simulink model "hvac_maborrelli_singapur_nzones_TCH"  (R2021a)
settings: Solver=ode45  StartTime=0.0  StopTime=Inf  FixedStep=2  RelTol=1e-3  EnableMultiTasking=on
values from neighbouring files (symbols this model uses):
  beta = 0.15    [main_td3_nzones.m]
  ci = ci'    [localResetFcn.m]    (also in localResetFcnT.m)
  CO2_max = 1200*1e-6    (= 0.0012)    [main_td3_nzones.m]
  high = 25    [main_td3_nzones.m]    (also in reward.m)
  low = -10    [isDone.m]    (also in main_td3_nzones.m = 22; reward.m = 22)
  params = params1    [main_td3_nzones.m]
  paramsnz =     [values4z_tch.mat]
  Ts = delta*Tr+(1-delta)*Toa + DT + DTH    [dynamics_hvac_maborrelli_singapur_1zone_tch.m]    (also in main_td3_nzones.m = 60)
  Ts2 = 900    [main.m]    (also in main_td3_nzones.m = 600)
undefined symbols (not defined in the file or in its folder): id, rl
libraries: simulink x15, dspmathops x5, rllib x1
settings Model: Creator=User  LastModifiedBy=Richi
settings SolverCC: AlgebraicLoopSolver=TrustRegion
settings DataIOCC: LimitDataPoints=on  SaveFormat=Array  SignalLoggingSaveFormat=ModelDataLogs
settings OptimizationCC: LifeSpan=inf
settings DebuggingCC: SolverPrmCheckMsg=warning  MultiTaskDSMMsg=warning  MultiTaskCondExecSysMsg=none  MultiTaskRateTransMsg=warning  StrictBusMsg=ErrorOnBusTreatedAsVector  SFUnexpectedBacktrackingDiag=warning  SFNoUnconditionalDefaultTransitionDiag=warning  SFExecutionAtInitializationDiag=none  SFMachineParentedDataDiag=warning  ArithmeticOperatorsInVariantConditions=warning
settings HardwareCC: ProdBitPerPointer=32  ProdBitPerSizeT=32  ProdBitPerPtrDiffT=32  ProdLargestAtomicFloat=None  ProdIntDivRoundTo=Undefined  ProdEndianess=Unspecified  ProdWordSize=32  ProdHWDeviceType=32-bit Generic
settings ModelReferenceCC: PropagateSignalLabelsOutOfModel=off
settings SFSimCC: SimUseLocalCustomCode=off  CustomCodeUndefinedFunction=UseInterfaceOnly
settings RTWCC: RTWUseLocalCustomCode=off
settings CodeAppCC: StateflowObjectComments=on
settings GRTTargetCC: TargetLangStandard=C89/C90 (ANSI)
settings ConfigComp: CovMetricSettings=dw  CovSaveCumulativeToWorkspaceVar=on  CovSaveSingleToWorkspaceVar=on  CovExternalEMLEnable=off

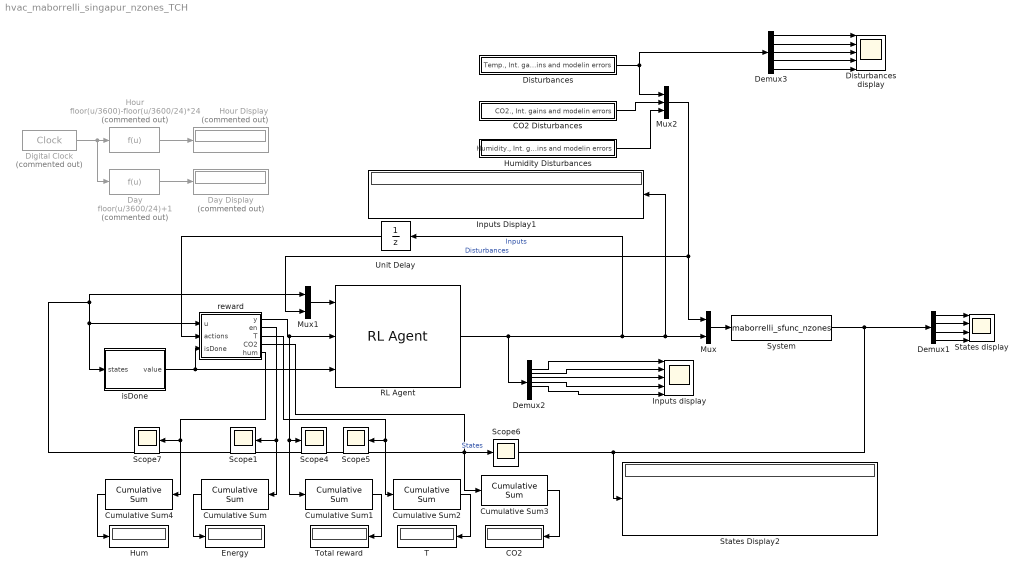
== system hvac_maborrelli_singapur_nzones_TCH ==
  CO2 : Display
  CO2 Disturbances : Subsystem  TreatAsAtomicUnit=on
  Cumulative Sum{,1..4} (5 alike) : dspmathops/Cumulative Sum  dim=Channels (running sum)  InputProcessing=Columns as channels (frame based)  reset_popup=None  roundingMode=Floor  overflowMode=off  outputDataTypeStr=Inherit: Same as accumulator  outputMin=[]  outputMax=[]  outputLastDataTypeStr=Inherit: Same as accumulator
  Day : Fcn  Commented=on  Expr=floor(u/3600/24)+1  SampleTime=1800
  Day Display : Display  Commented=on
  Demux1 : Demux
  Demux2 : Demux  Outputs=6
  Demux3 : Demux  Outputs=5
  Digital Clock : DigitalClock  Commented=on  SampleTime=60
  Disturbances : Subsystem  TreatAsAtomicUnit=on
  Disturbances display : Scope  NumInputPorts=5
  Energy : Display
  Hour : Fcn  Commented=on  Expr=floor(u/3600)-floor(u/3600/24)*24  SampleTime=1800
  Hour Display : Display  Commented=on
  Hum : Display
  Humidity Disturbances : Subsystem  TreatAsAtomicUnit=on
  Inputs Display1 : Display
  Inputs display : Scope  NumInputPorts=5
  Mux : Mux  Inputs=2
  Mux1 : Mux  Inputs=2
  Mux2 : Mux  Inputs=3
  RL Agent : rllib/RL Agent  Agent=rl.util.PolicyInstance.get('hvac_maborrelli_singapur_nzones_with_MPC_v3_manualdist_3/RL Agent')  ExternalActionAsInput=off  ProvideCumRwd=off  TreatAsDirectFeedthrough=on
  Scope{1,4..7} (5 alike) : Scope
  States Display2 : Display
  States display : Scope  NumInputPorts=4
  System : S-Function  FunctionName=maborrelli_sfunc_nzones  Parameters=ci,paramsnz,Ts  SFunctionDeploymentMode=off  EnableBusSupport=off
  T : Display
  Total reward : Display
  Unit Delay : UnitDelay  SampleTime=Ts2  HasFrameUpgradeWarning=on
  isDone : MATLAB Function  TreatAsAtomicUnit=on
  reward : MATLAB Function  TreatAsAtomicUnit=on
  wires:
  Mux/1 -> System/1
  System/1 -> Demux1/1, States Display2/1, Mux1/1, isDone/1(states), reward/1(u)  "States"
  RL Agent/1 -> Unit Delay/1, Mux/2, Inputs Display1/1, Demux2/1  "Inputs"
  Hour/1 -> Hour Display/1
  Digital Clock/1 -> Day/1, Hour/1
  Day/1 -> Day Display/1
  Demux1/1 -> States display/1
  Demux1/2 -> States display/2
  Demux1/3 -> States display/3
  Demux1/4 -> States display/4
  Demux2/1 -> Inputs display/1
  Demux2/2 -> Inputs display/2
  Demux2/3 -> Inputs display/3
  Demux2/4 -> Inputs display/4
  Demux2/5 -> Inputs display/5
  isDone/1(value) -> reward/3(isDone), RL Agent/3
  Mux1/1 -> RL Agent/1
  Unit Delay/1 -> reward/2(actions)
  Disturbances/1("Temp., Int. gains and modelin errors") -> Mux2/1, Demux3/1
  CO2 Disturbances/1("CO2., Int. gains and modelin errors") -> Mux2/2
  Humidity Disturbances/1("Humidity., Int. gains and modelin errors") -> Mux2/3
  Mux2/1 -> Mux1/2, Mux/1  "Disturbances"
  Demux3/1 -> Disturbances display/1
  Cumulative Sum4/1 -> Hum/1
  reward/4(CO2) -> Cumulative Sum3/1, Scope6/1
  Cumulative Sum/1 -> Energy/1
  Cumulative Sum2/1 -> T/1
  reward/5(hum) -> Cumulative Sum4/1, Scope7/1
  Cumulative Sum3/1 -> CO2/1
  reward/1(y) -> Cumulative Sum1/1, Scope4/1, RL Agent/2
  reward/3(T) -> Cumulative Sum2/1, Scope5/1
  Cumulative Sum1/1 -> Total reward/1
  reward/2(en) -> Cumulative Sum/1, Scope1/1
  Demux3/2 -> Disturbances display/2
  Demux3/3 -> Disturbances display/3
  Demux3/4 -> Disturbances display/4
  Demux3/5 -> Disturbances display/5

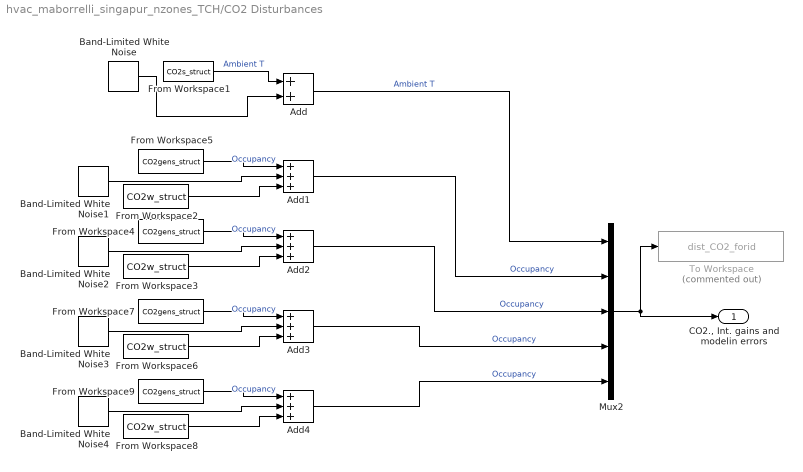
== system hvac_maborrelli_singapur_nzones_TCH/CO2 Disturbances ==
  Add : Sum
  Add{1..4} (4 alike) : Sum  Inputs=+++
  Band-Limited White Noise{,1..4} (5 alike) : simulink/Sources/Band-Limited White Noise  Cov=0  Ts=Ts  seed=[23341]
  From Workspace1 : FromWorkspace  VariableName=CO2s_struct  OutDataTypeStr=double  SampleTime=Ts  ZeroCross=off
  From Workspace{2..3,6,8} (4 alike) : FromWorkspace  VariableName=CO2w_struct  OutDataTypeStr=double  SampleTime=Ts  ZeroCross=off
  From Workspace{4..5,7,9} (4 alike) : FromWorkspace  VariableName=CO2gens_struct  OutDataTypeStr=double  SampleTime=Ts  ZeroCross=off
  Mux2 : Mux  Inputs=5
  To Workspace : ToWorkspace  Commented=on  VariableName=dist_CO2_forid  SaveFormat=Timeseries  SampleTime=id.Delta
  "CO2., Int. gains and modelin errors" : Outport
  wires:
  From Workspace1/1 -> Add/1  "Ambient T"
  Band-Limited White Noise/1 -> Add/2
  Add/1 -> Mux2/1  "Ambient T"
  From Workspace5/1 -> Add1/1  "Occupancy"
  Band-Limited White Noise1/1 -> Add1/2
  From Workspace2/1 -> Add1/3
  Mux2/1 -> "CO2., Int. gains and modelin errors"/1, To Workspace/1
  Add1/1 -> Mux2/2  "Occupancy"
  Add2/1 -> Mux2/3  "Occupancy"
  From Workspace3/1 -> Add2/3
  Band-Limited White Noise2/1 -> Add2/2
  From Workspace4/1 -> Add2/1  "Occupancy"
  Add3/1 -> Mux2/4  "Occupancy"
  From Workspace6/1 -> Add3/3
  Band-Limited White Noise3/1 -> Add3/2
  From Workspace7/1 -> Add3/1  "Occupancy"
  Add4/1 -> Mux2/5  "Occupancy"
  From Workspace8/1 -> Add4/3
  Band-Limited White Noise4/1 -> Add4/2
  From Workspace9/1 -> Add4/1  "Occupancy"

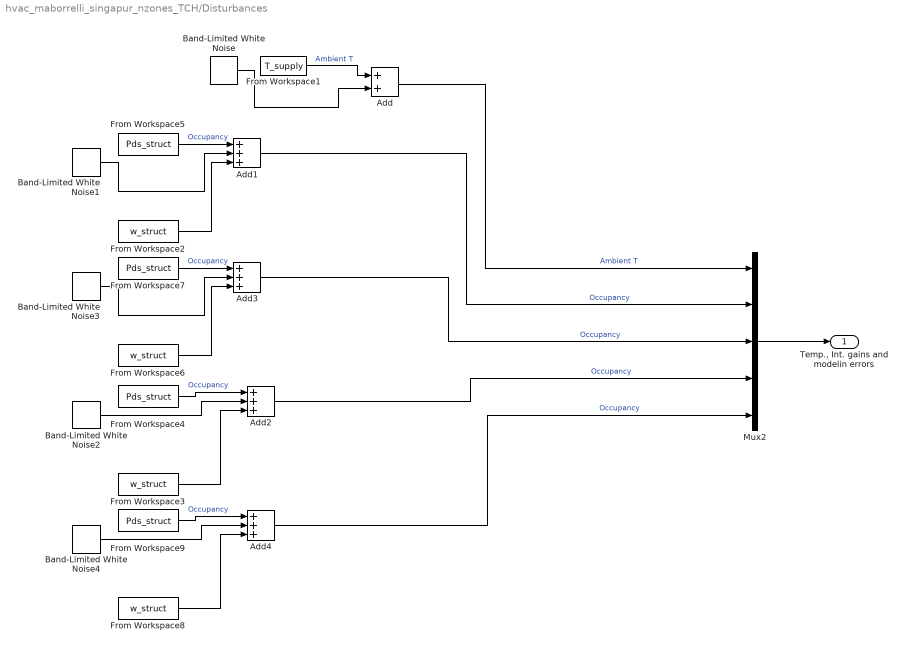
== system hvac_maborrelli_singapur_nzones_TCH/Disturbances ==
  Add : Sum
  Add{1..4} (4 alike) : Sum  Inputs=+++
  Band-Limited White Noise{,1..4} (5 alike) : simulink/Sources/Band-Limited White Noise  Cov=0  Ts=Ts2  seed=[23341]
  From Workspace1 : FromWorkspace  VariableName=T_supply  OutDataTypeStr=double  SampleTime=Ts  ZeroCross=off
  From Workspace{2..3,6,8} (4 alike) : FromWorkspace  VariableName=w_struct  OutDataTypeStr=double  SampleTime=Ts  ZeroCross=off
  From Workspace{4..5,7,9} (4 alike) : FromWorkspace  VariableName=Pds_struct  OutDataTypeStr=double  SampleTime=Ts  ZeroCross=off
  Mux2 : Mux  Inputs=5
  "Temp., Int. gains and modelin errors" : Outport
  wires:
  Add1/1 -> Mux2/2  "Occupancy"
  From Workspace1/1 -> Add/1  "Ambient T"
  Band-Limited White Noise/1 -> Add/2
  Add/1 -> Mux2/1  "Ambient T"
  From Workspace5/1 -> Add1/1  "Occupancy"
  Band-Limited White Noise1/1 -> Add1/2
  From Workspace2/1 -> Add1/3
  Mux2/1 -> "Temp., Int. gains and modelin errors"/1
  Add2/1 -> Mux2/4  "Occupancy"
  Band-Limited White Noise2/1 -> Add2/2
  From Workspace3/1 -> Add2/3
  Add3/1 -> Mux2/3  "Occupancy"
  Band-Limited White Noise3/1 -> Add3/2
  From Workspace6/1 -> Add3/3
  From Workspace7/1 -> Add3/1  "Occupancy"
  From Workspace4/1 -> Add2/1  "Occupancy"
  Add4/1 -> Mux2/5  "Occupancy"
  From Workspace8/1 -> Add4/3
  From Workspace9/1 -> Add4/1  "Occupancy"
  Band-Limited White Noise4/1 -> Add4/2

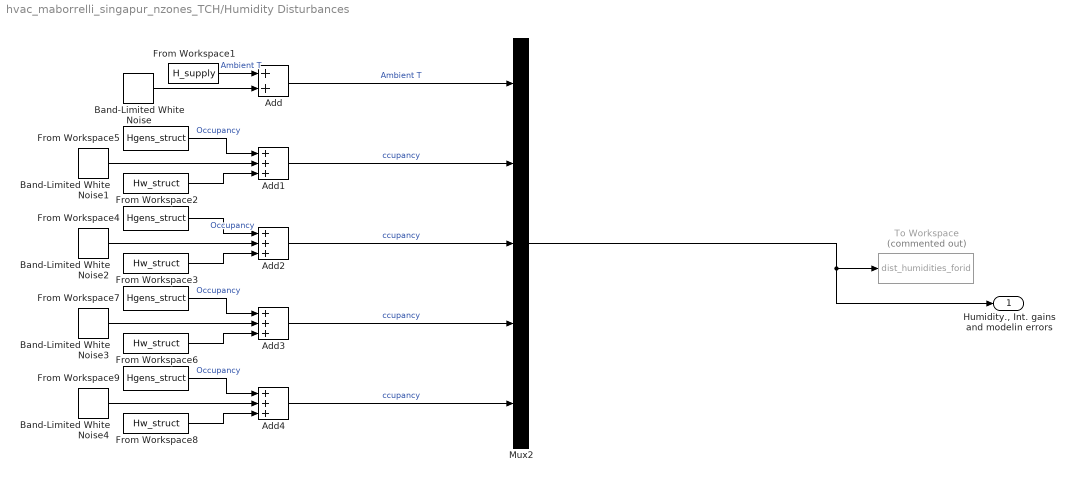
== system hvac_maborrelli_singapur_nzones_TCH/Humidity Disturbances ==
  Add : Sum
  Add{1..4} (4 alike) : Sum  Inputs=+++
  Band-Limited White Noise{,1..4} (5 alike) : simulink/Sources/Band-Limited White Noise  Cov=0  Ts=Ts  seed=[23341]
  From Workspace1 : FromWorkspace  VariableName=H_supply  OutDataTypeStr=double  SampleTime=Ts  ZeroCross=off
  From Workspace{2..3,6,8} (4 alike) : FromWorkspace  VariableName=Hw_struct  OutDataTypeStr=double  SampleTime=Ts  ZeroCross=off
  From Workspace{4..5,7,9} (4 alike) : FromWorkspace  VariableName=Hgens_struct  OutDataTypeStr=double  SampleTime=Ts  ZeroCross=off
  Mux2 : Mux  Inputs=5
  To Workspace : ToWorkspace  Commented=on  VariableName=dist_humidities_forid  SaveFormat=Timeseries  SampleTime=id.Delta
  "Humidity., Int. gains and modelin errors" : Outport
  wires:
  From Workspace1/1 -> Add/1  "Ambient T"
  Band-Limited White Noise/1 -> Add/2
  Add/1 -> Mux2/1  "Ambient T"
  From Workspace5/1 -> Add1/1  "Occupancy"
  Band-Limited White Noise1/1 -> Add1/2
  From Workspace2/1 -> Add1/3
  Mux2/1 -> "Humidity., Int. gains and modelin errors"/1, To Workspace/1
  Add1/1 -> Mux2/2  "ccupancy"
  Add2/1 -> Mux2/3  "ccupancy"
  From Workspace3/1 -> Add2/3
  From Workspace4/1 -> Add2/1  "Occupancy"
  Band-Limited White Noise2/1 -> Add2/2
  Add3/1 -> Mux2/4  "ccupancy"
  From Workspace6/1 -> Add3/3
  From Workspace7/1 -> Add3/1  "Occupancy"
  Band-Limited White Noise3/1 -> Add3/2
  Add4/1 -> Mux2/5  "ccupancy"
  From Workspace8/1 -> Add4/3
  From Workspace9/1 -> Add4/1  "Occupancy"
  Band-Limited White Noise4/1 -> Add4/2

== matlab function hvac_maborrelli_singapur_nzones_TCH/isDone ==
  data: states input; value output
function value = isDone(states)
 low = -0;
 max = 50;
 value = 0; 
 %disp(length(block.InputPort(1).Data))
 for i=1:length(states)
     %disp(i)
     if i <=4
        aux = states(i);
        if (aux < low || aux > max) 
            %disp(abs(aux - low))
            value = 1;
            break
        end
     elseif i>=9 && i<=12
        if states(i)>(3200*1e-6)
            value = 1;
            break
        end
     end
 end

== matlab function hvac_maborrelli_singapur_nzones_TCH/reward ==
  data: u input; y output; actions input; isDone input; en output; T output; CO2 output; hum output; low parameter; high parameter; beta parameter; params parameter; CO2_max parameter
function [y, en, T,  CO2, hum] = reward(u ,  actions, isDone, low, high, beta, params, CO2_max)
 reward = 0;
 cp = params.cp;
 eta = params.eta;
 kf = params.kf;
 eta_h = params.eta_h;
 nz = 4;
 ms = actions(1:nz);
 Dt = actions(nz+1);
 Dth = actions(nz+2:2*nz+1);
 delta = actions(2*nz + 2);
 T_in = u(1:nz);
 CO2_in = u(2*nz+1:3*nz);
 hum_in = u(4*nz+1:5*nz);
 %Se inician las metricas
 CO2 = 0; hum = 0;T = 0;
 %Añadir energía:
 e = (kf*sum((ms).^2))/1000;
 e = e + ((-cp/eta)*sum(ms)*(Dt))/1000;
 for i=1:nz
     %Se aplica la penalización por energía al usar la calefacción
     if Dth(i) ~= 0
         e = e + ((cp/eta_h)*ms(i)*(Dth(i) - Dt))/1000;
     end
     %Se penaliza si hay calefacción pero no flujo de aire.
     if ms(i) == 0 && Dth(i)~=0
         reward = reward - 10;
     end
     %Se penaliza si hay enfriamiento pero no flujo de aire.
     if ms(i) == 0 && Dt~=0
         reward = reward - 0.5;
     end
     %Se penaliza romper las restricciones de temperatura.
     aux = T_in(i);
     if (aux < low || aux > high)
        T = 0.5*(min(abs(aux - low), abs(aux - high))+ (min( abs(aux - low), abs(aux - high)))^2);
        reward = reward - T;
     end
     %Se penaliza romper las restricciones de concentración de CO2
     aux_co2 = CO2_in(i);
     if CO2_max < aux_co2
        %disp(-abs(CO2_max - u(3))*10000)
        CO2 = abs(CO2_max - aux_co2)*10000;
        reward = reward - CO2;
     end
     %Se penaliza romper las restricciones de humedad.
     Hum = hum_in(i);
     if (0.35 > Hum) || (Hum > 0.65)
         hum = min(abs(Hum-0.35),abs(Hum-0.65));
         reward = reward - hum;
         %disp(min(abs(Hum-0.35),abs(Hum-0.65))*7)
     end
     %Entregar bonificación por estar en el estado
     %if (aux >= low && aux <= high)
     %    reward = reward + 1;
     %end
 %Se aplica el peso a la energía
 reward = reward -beta* e; 
 en = e;
 end
 if isDone
     reward = -2000;
 end
y = reward;
